simulink model "RoboticArm"  (R2023b)
settings: Solver=ode23t  StartTime=0.0  StopTime=100  RelTol=1e-3
model workspace: external: MATLAB File D:\Projects\RoboticArm\RoboticArm_DataFile1.m (data not in the file)
undefined symbols (not defined in the file or in its folder): dfdbk, dFilt, nfdbk, nFilt, smiData, ST, X, Y, Z
libraries: sm_lib x180, fl_lib x129, nesl_utility x69, ee_lib x39, slpidlib x25, simulink x18, SignalEditorBlockLib x1
(part 3 of 7)

== system RoboticArm/Control System3/Subsystem3 ==
  signal : Inport
  Abs : Abs  SaturateOnIntegerOverflow=off
  Fcn : Fcn  Expr=u(1)<0
  Gain : Gain  Gain=5
  "[0...5]" : Saturate  UpperLimit=5  LowerLimit=0
  duty : Outport
  rev : Outport  Port=2
  wires:
  signal/1 -> Fcn/1, Abs/1
  Abs/1 -> "[0...5]"/1
  Fcn/1 -> Gain/1
  Gain/1 -> rev/1
  "[0...5]"/1 -> duty/1

== system RoboticArm/Control System3/Subsystem4 ==
  signal : Inport
  Abs : Abs  SaturateOnIntegerOverflow=off
  Fcn : Fcn  Expr=u(1)<0
  Gain : Gain  Gain=5
  "[0...5]" : Saturate  UpperLimit=5  LowerLimit=0
  duty : Outport
  rev : Outport  Port=2
  wires:
  "[0...5]"/1 -> duty/1
  Gain/1 -> rev/1
  Fcn/1 -> Gain/1
  Abs/1 -> "[0...5]"/1
  signal/1 -> Abs/1, Fcn/1

== system RoboticArm/Control System3/Subsystem5 ==
  signal : Inport
  Abs : Abs  SaturateOnIntegerOverflow=off
  Fcn : Fcn  Expr=u(1)<0
  Gain : Gain  Gain=5
  "[0...5]" : Saturate  UpperLimit=5  LowerLimit=0
  duty : Outport
  rev : Outport  Port=2
  wires:
  signal/1 -> Fcn/1, Abs/1
  Abs/1 -> "[0...5]"/1
  Fcn/1 -> Gain/1
  Gain/1 -> rev/1
  "[0...5]"/1 -> duty/1

== system RoboticArm/Control System3/Subsystem6 ==
  signal : Inport
  Abs : Abs  SaturateOnIntegerOverflow=off
  Fcn : Fcn  Expr=u(1)<0
  Gain : Gain  Gain=5
  "[0...5]" : Saturate  UpperLimit=5  LowerLimit=0
  duty : Outport
  rev : Outport  Port=2
  wires:
  "[0...5]"/1 -> duty/1
  Gain/1 -> rev/1
  Fcn/1 -> Gain/1
  Abs/1 -> "[0...5]"/1
  signal/1 -> Abs/1, Fcn/1

== system RoboticArm/Control System3/Transfer Function ==
  Fdbk : Inport
  Bus Creator6 : BusCreator  Inputs=6
  Bus Selector2 : BusSelector  OutputSignals=tAngle,bAngle,fAngle,wAngle,hAngle,gAngle
  Constant1 : Constant  Value=pi/2
  Discrete Transfer Fcn{,1..5} (6 alike) : DiscreteTransferFcn  Numerator=nFilt  Denominator=dFilt  SampleTime=ST
  Sum1 : Sum  Inputs=|+-
  Angles : Outport
  wires:
  Sum1/1 -> Discrete Transfer Fcn1/1
  Discrete Transfer Fcn2/1 -> Bus Creator6/3  "fAngle"
  Discrete Transfer Fcn/1 -> Bus Creator6/1  "tAngle"
  Discrete Transfer Fcn3/1 -> Bus Creator6/4  "wAngle"
  Discrete Transfer Fcn4/1 -> Bus Creator6/5  "hAngle"
  Fdbk/1 -> Bus Selector2/1
  Discrete Transfer Fcn5/1 -> Bus Creator6/6  "gAngle"
  Discrete Transfer Fcn1/1 -> Bus Creator6/2  "bAngle"
  Constant1/1 -> Sum1/2
  Bus Selector2/2 -> Sum1/1  "<bAngle>"
  Bus Selector2/4 -> Discrete Transfer Fcn3/1  "<wAngle>"
  Bus Selector2/1 -> Discrete Transfer Fcn/1  "<tAngle>"
  Bus Creator6/1 -> Angles/1
  Bus Selector2/3 -> Discrete Transfer Fcn2/1  "<fAngle>"
  Bus Selector2/6 -> Discrete Transfer Fcn5/1  "<gAngle>"
  Bus Selector2/5 -> Discrete Transfer Fcn4/1  "<hAngle>"

== system RoboticArm/Controller1/Signal Conditioning ==
  note: Anti-aliasing filters
  fddk : Inport
  Bus Creator3 : BusCreator  Inputs=6
  Bus Selector : BusSelector  OutputSignals=tAngle,bAngle,fAngle,wAngle,hAngle,gAngle
  Discrete Transfer Fcn{,1..5} (6 alike) : DiscreteTransferFcn  Numerator=nFilt  Denominator=dFilt  SampleTime=ST
  IC : Constant  Value=pi
  Sum : Sum  Inputs=|+-
  angles (rad) : Outport  VectorParamsAs1DForOutWhenUnconnected=off
  wires:
  IC/1 -> Sum/2
  Sum/1 -> Discrete Transfer Fcn1/1
  Bus Selector/2 -> Sum/1  "<bAngle>"
  Bus Selector/6 -> Discrete Transfer Fcn5/1  "<gAngle>"
  Bus Selector/5 -> Discrete Transfer Fcn4/1  "<hAngle>"
  Discrete Transfer Fcn5/1 -> Bus Creator3/6  "gAngle"
  Discrete Transfer Fcn4/1 -> Bus Creator3/5  "hAngle"
  Bus Creator3/1 -> angles (rad)/1
  Discrete Transfer Fcn3/1 -> Bus Creator3/4  "wAngle"
  Discrete Transfer Fcn2/1 -> Bus Creator3/3  "fAngle"
  Bus Selector/3 -> Discrete Transfer Fcn2/1  "<fAngle>"
  Bus Selector/4 -> Discrete Transfer Fcn3/1  "<wAngle>"
  Bus Selector/1 -> Discrete Transfer Fcn/1  "<tAngle>"
  fddk/1 -> Bus Selector/1
  Discrete Transfer Fcn/1 -> Bus Creator3/1  "tAngle"
  Discrete Transfer Fcn1/1 -> Bus Creator3/2  "bAngle"

== system RoboticArm/Controller1/bicepCMD ==
  Vcmd : Inport
  Vbrk : Inport  Port=2
  Abs : Abs  SaturateOnIntegerOverflow=off
  Fcn : Fcn  Expr=u(1)<0
  Gain : Gain  Gain=5
  "[0...5]" : Saturate  UpperLimit=100  LowerLimit=0
  "[0...5] " : Saturate  UpperLimit=5  LowerLimit=0
  Duty : Outport  VectorParamsAs1DForOutWhenUnconnected=off
  REV : Outport  Port=2  VectorParamsAs1DForOutWhenUnconnected=off
  BRK : Outport  Port=3  VectorParamsAs1DForOutWhenUnconnected=off
  wires:
  "[0...5] "/1 -> BRK/1
  Vbrk/1 -> "[0...5] "/1
  Vcmd/1 -> Fcn/1, Abs/1
  Abs/1 -> "[0...5]"/1
  Fcn/1 -> Gain/1
  "[0...5]"/1 -> Duty/1
  Gain/1 -> REV/1

== system RoboticArm/Controller1/forearmCMD ==
  Vcmd : Inport
  Vbrk : Inport  Port=2
  Abs : Abs  SaturateOnIntegerOverflow=off
  Fcn : Fcn  Expr=u(1)<0
  Gain : Gain  Gain=5
  "[0...5]" : Saturate  UpperLimit=5  LowerLimit=0
  "[0...5] " : Saturate  UpperLimit=5  LowerLimit=0
  Duty : Outport  VectorParamsAs1DForOutWhenUnconnected=off
  REV : Outport  Port=2  VectorParamsAs1DForOutWhenUnconnected=off
  BRK : Outport  Port=3  VectorParamsAs1DForOutWhenUnconnected=off
  wires:
  Gain/1 -> REV/1
  "[0...5]"/1 -> Duty/1
  Fcn/1 -> Gain/1
  Abs/1 -> "[0...5]"/1
  Vcmd/1 -> Abs/1, Fcn/1
  Vbrk/1 -> "[0...5] "/1
  "[0...5] "/1 -> BRK/1

== system RoboticArm/Controller1/gripperCMD ==
  Vcmd : Inport
  Vbrk : Inport  Port=2
  Abs : Abs  SaturateOnIntegerOverflow=off
  Fcn : Fcn  Expr=u(1)<0
  Gain : Gain  Gain=5
  "[0...5]" : Saturate  UpperLimit=5  LowerLimit=0
  "[0...5] " : Saturate  UpperLimit=5  LowerLimit=0
  Duty : Outport  VectorParamsAs1DForOutWhenUnconnected=off
  REV : Outport  Port=2  VectorParamsAs1DForOutWhenUnconnected=off
  BRK : Outport  Port=3  VectorParamsAs1DForOutWhenUnconnected=off
  wires:
  Gain/1 -> REV/1
  "[0...5]"/1 -> Duty/1
  Fcn/1 -> Gain/1
  Abs/1 -> "[0...5]"/1
  Vcmd/1 -> Abs/1, Fcn/1
  Vbrk/1 -> "[0...5] "/1
  "[0...5] "/1 -> BRK/1

== system RoboticArm/Controller1/handCMD ==
  Vcmd : Inport
  Vbrk : Inport  Port=2
  Abs : Abs  SaturateOnIntegerOverflow=off
  Fcn : Fcn  Expr=u(1)<0
  Gain : Gain  Gain=5
  "[0...5]" : Saturate  UpperLimit=5  LowerLimit=0
  "[0...5] " : Saturate  UpperLimit=5  LowerLimit=0
  Duty : Outport  VectorParamsAs1DForOutWhenUnconnected=off
  REV : Outport  Port=2  VectorParamsAs1DForOutWhenUnconnected=off
  BRK : Outport  Port=3  VectorParamsAs1DForOutWhenUnconnected=off
  wires:
  "[0...5] "/1 -> BRK/1
  Vbrk/1 -> "[0...5] "/1
  Vcmd/1 -> Fcn/1, Abs/1
  Abs/1 -> "[0...5]"/1
  Fcn/1 -> Gain/1
  "[0...5]"/1 -> Duty/1
  Gain/1 -> REV/1

== system RoboticArm/Controller1/turntableCMD ==
  Vcmd : Inport
  Vbrk : Inport  Port=2
  Abs : Abs  SaturateOnIntegerOverflow=off
  Fcn : Fcn  Expr=u(1)<0
  Gain : Gain  Gain=5
  "[0...5]" : Saturate  UpperLimit=5  LowerLimit=0
  "[0...5] " : Saturate  UpperLimit=5  LowerLimit=0
  Duty : Outport  VectorParamsAs1DForOutWhenUnconnected=off
  REV : Outport  Port=2  VectorParamsAs1DForOutWhenUnconnected=off
  BRK : Outport  Port=3  VectorParamsAs1DForOutWhenUnconnected=off
  wires:
  Gain/1 -> REV/1
  "[0...5]"/1 -> Duty/1
  Fcn/1 -> Gain/1
  Abs/1 -> "[0...5]"/1
  Vcmd/1 -> Abs/1, Fcn/1
  Vbrk/1 -> "[0...5] "/1
  "[0...5] "/1 -> BRK/1

== system RoboticArm/Controller1/wristCMD ==
  Vcmd : Inport
  Vbrk : Inport  Port=2
  Abs : Abs  SaturateOnIntegerOverflow=off
  Fcn : Fcn  Expr=u(1)<0
  Gain : Gain  Gain=5
  "[0...5]" : Saturate  UpperLimit=5  LowerLimit=0
  "[0...5] " : Saturate  UpperLimit=5  LowerLimit=0
  Duty : Outport  VectorParamsAs1DForOutWhenUnconnected=off
  REV : Outport  Port=2  VectorParamsAs1DForOutWhenUnconnected=off
  BRK : Outport  Port=3  VectorParamsAs1DForOutWhenUnconnected=off
  wires:
  Gain/1 -> REV/1
  "[0...5]"/1 -> Duty/1
  Fcn/1 -> Gain/1
  Abs/1 -> "[0...5]"/1
  Vcmd/1 -> Abs/1, Fcn/1
  Vbrk/1 -> "[0...5] "/1
  "[0...5] "/1 -> BRK/1

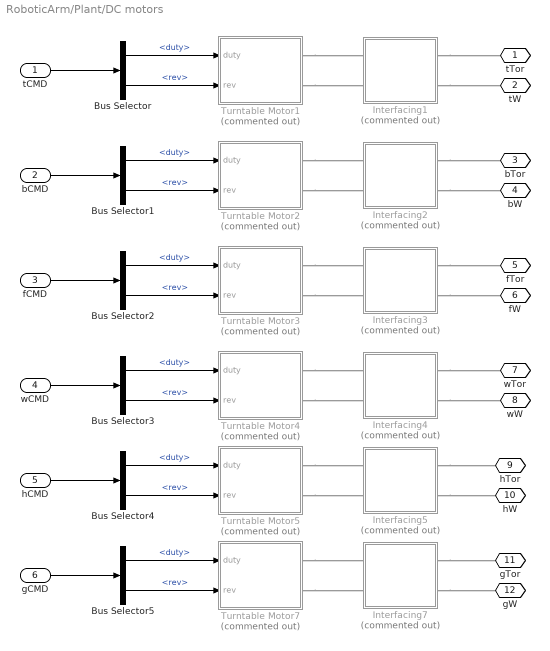
== system RoboticArm/Plant/DC motors ==
  tCMD : Inport
  bCMD : Inport  Port=2
  fCMD : Inport  Port=3
  wCMD : Inport  Port=4
  hCMD : Inport  Port=5
  gCMD : Inport  Port=6
  Bus Selector{,1..5} (6 alike) : BusSelector  OutputSignals=duty,rev
  Interfacing1 : Subsystem  Commented=on
      mask Display: image('interface-4.png');
  Interfacing2 : Subsystem  Commented=on
      mask Display: image('interface-4.png');
  Interfacing3 : Subsystem  Commented=on
      mask Display: image('interface-4.png');
  Interfacing4 : Subsystem  Commented=on
      mask Display: image('interface-4.png');
  Interfacing5 : Subsystem  Commented=on
      mask Display: image('interface-4.png');
  Interfacing7 : Subsystem  Commented=on
      mask Display: image('interface-4.png');
  Turntable Motor1 : Subsystem  Commented=on
      mask Display: image('servo1.jpg');
  Turntable Motor2 : Subsystem  Commented=on
      mask Display: image('servo1.jpg');
  Turntable Motor3 : Subsystem  Commented=on
      mask Display: image('servo1.jpg');
  Turntable Motor4 : Subsystem  Commented=on
      mask Display: image('servo1.jpg');
  Turntable Motor5 : Subsystem  Commented=on
      mask Display: image('servo1.jpg');
  Turntable Motor7 : Subsystem  Commented=on
      mask Display: image('servo1.jpg');
  tTor : PMIOPort  Side=Right
  tW : PMIOPort  Port=2  Side=Right
  bTor : PMIOPort  Port=3  Side=Right
  bW : PMIOPort  Port=4  Side=Right
  fTor : PMIOPort  Port=5  Side=Right
  fW : PMIOPort  Port=6  Side=Right
  wTor : PMIOPort  Port=7  Side=Right
  wW : PMIOPort  Port=8  Side=Right
  hTor : PMIOPort  Port=9  Side=Right
  hW : PMIOPort  Port=10  Side=Right
  gTor : PMIOPort  Port=11  Side=Right
  gW : PMIOPort  Port=12  Side=Right
  wires:
  wCMD/1 -> Bus Selector3/1
  bCMD/1 -> Bus Selector1/1
  gCMD/1 -> Bus Selector5/1
  fCMD/1 -> Bus Selector2/1
  tCMD/1 -> Bus Selector/1
  hCMD/1 -> Bus Selector4/1
  Bus Selector/1 -> Turntable Motor1/1(duty)  "<duty>"
  Bus Selector/2 -> Turntable Motor1/2(rev)  "<rev>"
  Bus Selector1/1 -> Turntable Motor2/1(duty)  "<duty>"
  Bus Selector1/2 -> Turntable Motor2/2(rev)  "<rev>"
  Bus Selector2/2 -> Turntable Motor3/2(rev)  "<rev>"
  Bus Selector2/1 -> Turntable Motor3/1(duty)  "<duty>"
  Bus Selector3/1 -> Turntable Motor4/1(duty)  "<duty>"
  Bus Selector3/2 -> Turntable Motor4/2(rev)  "<rev>"
  Bus Selector4/1 -> Turntable Motor5/1(duty)  "<duty>"
  Bus Selector4/2 -> Turntable Motor5/2(rev)  "<rev>"
  Bus Selector5/1 -> Turntable Motor7/1(duty)  "<duty>"
  Bus Selector5/2 -> Turntable Motor7/2(rev)  "<rev>"
  connections:
  Interfacing1/RConn2 -- tW/RConn1
  Interfacing1/RConn1 -- tTor/RConn1
  Interfacing2/RConn1 -- bTor/RConn1
  Interfacing2/RConn2 -- bW/RConn1
  Interfacing3/RConn2 -- fW/RConn1
  Interfacing3/RConn1 -- fTor/RConn1
  Interfacing4/RConn1 -- wTor/RConn1
  Interfacing4/RConn2 -- wW/RConn1
  Interfacing5/RConn2 -- hW/RConn1
  Interfacing5/RConn1 -- hTor/RConn1
  Interfacing7/RConn1 -- gTor/RConn1
  Interfacing7/RConn2 -- gW/RConn1
  Turntable Motor1/RConn2 -- Interfacing1/LConn2
  Turntable Motor1/RConn1 -- Interfacing1/LConn1
  Turntable Motor2/RConn1 -- Interfacing2/LConn1
  Turntable Motor2/RConn2 -- Interfacing2/LConn2
  Turntable Motor3/RConn2 -- Interfacing3/LConn2
  Turntable Motor3/RConn1 -- Interfacing3/LConn1
  Turntable Motor4/RConn1 -- Interfacing4/LConn1
  Turntable Motor4/RConn2 -- Interfacing4/LConn2
  Turntable Motor5/RConn2 -- Interfacing5/LConn2
  Turntable Motor5/RConn1 -- Interfacing5/LConn1
  Turntable Motor7/RConn1 -- Interfacing7/LConn1
  Turntable Motor7/RConn2 -- Interfacing7/LConn2

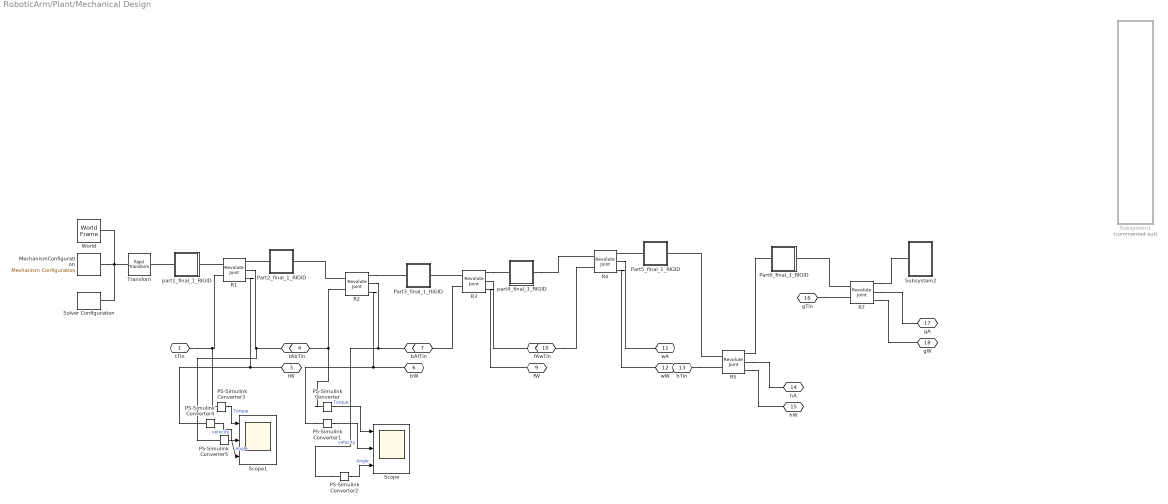
== system RoboticArm/Plant/Mechanical Design ==
  MechanismConfiguration : sm_lib/Utilities/Mechanism Configuration  UniformGravity=Constant  GravityVector=[0 -9.81 0]  GravityVectorUnits=m/s^2  LinearizationDelta=0.001  JointModeTransitionNonlinearIterations=2
  PS-Simulink Converter{,1..5} (6 alike) : nesl_utility/PS-Simulink Converter  PhysicalDomain=network_engine_domain  SubClassName=ps_output  LeftPortType=input  RightPortType=output  PseudoPeriodic=off  Frequencies=[]  VectorFormat=inherit  Unit=inherit  AffineConversion=off
  Part2_final_1_RIGID : Subsystem
  Part3_final_1_RIGID : Subsystem
  Part5_final_1_RIGID : Subsystem
  Part6_final_1_RIGID : Subsystem
  R{1..5,7} (6 alike) : sm_lib/Joints/Revolute Joint  JointMode=Normal  SenseConstraintForce=off  SenseConstraintForceX=off  SenseConstraintForceY=off  SenseConstraintForceZ=off  SenseConstraintTorque=off  SenseConstraintTorqueX=off  SenseConstraintTorqueY=off  SenseConstraintTorqueZ=off  SenseTotalForce=off  SenseTotalForceX=off  SenseTotalForceY=off  SenseTotalForceZ=off  SenseTotalTorque=off  SenseTotalTorqueX=off  SenseTotalTorqueY=off  SenseTotalTorqueZ=off  CompositeWrenchDir=FollowerOnBase  CompositeWrenchFrame=BaseFrame  EquilibriumPosition=0  EquilibriumPositionUnits=rad  SpringStiffness=0  SpringStiffnessUnits=m*N/rad  DampingCoefficient=0  DampingCoefficientUnits=m*s*N/rad  TorqueActuationMode=InputTorque  MotionActuationMode=ComputedMotion  SensePosition=on  SenseVelocity=on  SenseAcceleration=off  SenseTorqueForce=off  SenseLowerLimitTorqueForce=off  SenseUpperLimitTorqueForce=off  LowerLimitSpecify=off  LowerLimitBound=-90  LowerLimitBoundUnits=deg  LowerLimitStiffness=1e4  LowerLimitStiffnessUnits=N*m/deg  LowerLimitDamping=10  LowerLimitDampingUnits=N*m/(deg/s)  LowerLimitTransitionRegionWidth=0.1  LowerLimitTransitionRegionWidthUnits=deg  UpperLimitSpecify=off  UpperLimitBound=90  UpperLimitBoundUnits=deg  UpperLimitStiffness=1e4  UpperLimitStiffnessUnits=N*m/deg  UpperLimitDamping=10  UpperLimitDampingUnits=N*m/(deg/s)  UpperLimitTransitionRegionWidth=0.1  UpperLimitTransitionRegionWidthUnits=deg  PositionTargetSpecify=on  PositionTargetPriority=High  PositionTargetValue=0  PositionTargetValueUnits=deg  VelocityTargetSpecify=on  VelocityTargetPriority=High  VelocityTargetValue=0  VelocityTargetValueUnits=deg/s
  Scope : Scope  NumInputPorts=3
  Scope1 : Scope  NumInputPorts=3
  Solver Configuration : nesl_utility/Solver Configuration  PhysicalDomain=network_engine_domain  SubClassName=solver  LeftPortType=input  RightPortType=generic  Tones=[]  Harmonics=[]  SimulateNoise=off  Profile=off  UseLocalSampling=off  EnableSwitchedLinearOptims=on  FrequencyDomain=off  UseCCode=off  RelTol=0.001  AbsTol=1e-06  MinStep=1e-09  ToWorkspace=off  RevertToSquareIcSolve=off  NumHomotopyIterations=100  PhasorMode=off  PhasorModeNumHarmonics=1  ConsistencySolver=NEWTON_FTOL  IndexReductionMethod=DerivativeReplacement  DoDC=off  ResidualTolerance=1e-09  ConsistencyTolSource=GLOBAL  ConsistencyAbsTol=0.001  ConsistencyRelTol=0.001  ConsistencyTolFactor=0.001  UseLocalSolver=off  LocalSolverChoice=NE_BACKWARD_EULER_ADVANCER  ResolveIndetEquations=on  FunctionEvalNumThread=1  LocalSolverSampleTime=0.001  DoFixedCost=off  MaxNonlinIter=3  MaxModeIter=2  ComputeImpulses=off  ImpulseIterations=2  LinearAlgebra=Sparse  LinearAlgebraNumThread=0  EquationFormulation=NE_TIME_EF  DelaysMemoryBudget=1024  AutomaticFiltering=on  FilteringTimeConstant=0.001  PartitionStorageMethod=AS_NEEDED  PartitionMemoryBudget=1024  PartitionMethod=FAST  MultibodyUseLocalSolver=off  MultibodyLocalSolverChoice=ODE1  MultibodyLocalSolverSampleTime=0.001
  Subsystem1 : Subsystem  Commented=on
  Subsystem2 : Subsystem
  Transforn : sm_lib/Frames and Transforms/Rigid Transform  TranslationMethod=None  TranslationStandardOffset=0  TranslationStandardOffsetUnits=m  TranslationStandardAxis=+Z  TranslationCartesianOffset=[0 0 0]  TranslationCartesianOffsetUnits=m  TranslationROffset=0  TranslationROffsetUnits=m  TranslationZOffset=0  TranslationZOffsetUnits=m  TranslationThetaOffset=0  TranslationThetaOffsetUnits=deg  RotationMethod=None  RotationAngleUnits=deg  RotationStandardAxis=+Z  RotationAngle=0.0  RotationArbitraryAxis=[0 0 1]  FollAlignAxisA=+X  BaseAlignAxisA=+Y  FollAlignAxisB=+Y  BaseAlignAxisB=+Z  RotationSequenceAxes=FollowerAxes  RotationSequence=XYX  RotationSequenceAngles=[0 0 0]  RotationSequenceAnglesUnits=deg  RotationMatrix=[1 0 0; 0 1 0; 0 0 1]  Quaternion=[1 0 0 0]
  World : sm_lib/Frames and Transforms/World Frame
  part1_final_1_RIGID : Subsystem
  part4_final_1_RIGID : Subsystem
  tTin : PMIOPort  Side=Left
  tA : PMIOPort  Port=2  Side=Right
  tW : PMIOPort  Port=3  Side=Left
  bTin : PMIOPort  Port=4  Side=Left
  bA : PMIOPort  Port=5  Side=Right
  bW : PMIOPort  Port=6  Side=Left
  fTin : PMIOPort  Port=7  Side=Left
  fA : PMIOPort  Port=8  Side=Right
  fW : PMIOPort  Port=9  Side=Left
  wTin : PMIOPort  Port=10  Side=Left
  wA : PMIOPort  Port=11  Side=Right
  wW : PMIOPort  Port=12  Side=Left
  hTin : PMIOPort  Port=13  Side=Left
  hA : PMIOPort  Port=14  Side=Right
  hW : PMIOPort  Port=15  Side=Left
  gTin : PMIOPort  Port=16  Side=Left
  gA : PMIOPort  Port=17  Side=Right
  gW : PMIOPort  Port=18  Side=Left
  wires:
  PS-Simulink Converter2/1 -> Scope/3  "Angle"
  PS-Simulink Converter5/1 -> Scope1/3  "Angle"
  PS-Simulink Converter/1 -> Scope/1  "Torque"
  PS-Simulink Converter4/1 -> Scope1/2  "velocity"
  PS-Simulink Converter1/1 -> Scope/2  "velocity"
  PS-Simulink Converter3/1 -> Scope1/1  "Torque"
  connections:
  R1/RConn2 -- tA/RConn1 -- PS-Simulink Converter5/LConn1
  PS-Simulink Converter1/LConn1 -- bW/RConn1 -- R2/RConn3
  PS-Simulink Converter/LConn1 -- bTin/RConn1 -- R2/LConn2
  R1/LConn2 -- tTin/RConn1 -- PS-Simulink Converter3/LConn1
  PS-Simulink Converter2/LConn1 -- bA/RConn1 -- R2/RConn2
  Solver Configuration/RConn1 -- World/RConn1 -- Transforn/LConn1 -- MechanismConfiguration/RConn1
  PS-Simulink Converter4/LConn1 -- tW/RConn1 -- R1/RConn3
  R7/RConn3 -- gW/RConn1
  R2/LConn1 -- Part2_final_1_RIGID/RConn1
  R5/RConn3 -- hW/RConn1
  R7/LConn1 -- Part6_final_1_RIGID/RConn1
  R5/RConn2 -- hA/RConn1
  wTin/RConn1 -- R4/LConn2
  R5/LConn1 -- Part5_final_1_RIGID/RConn1
  R3/RConn3 -- fW/RConn1
  R4/RConn3 -- wW/RConn1
  hTin/RConn1 -- R5/LConn2
  R3/LConn2 -- fTin/RConn1
  R7/RConn2 -- gA/RConn1
  R4/RConn2 -- wA/RConn1
  R3/RConn2 -- fA/RConn1
  gTin/RConn1 -- R7/LConn2
  Part2_final_1_RIGID/LConn1 -- R1/RConn1
  R7/RConn1 -- Subsystem2/LConn1
  R3/LConn1 -- Part3_final_1_RIGID/RConn1
  Part5_final_1_RIGID/LConn1 -- R4/RConn1
  part1_final_1_RIGID/LConn1 -- Transforn/RConn1
  R3/RConn1 -- part4_final_1_RIGID/LConn1
  part4_final_1_RIGID/RConn1 -- R4/LConn1
  R2/RConn1 -- Part3_final_1_RIGID/LConn1
  R1/LConn1 -- part1_final_1_RIGID/RConn1
  Part6_final_1_RIGID/LConn1 -- R5/RConn1

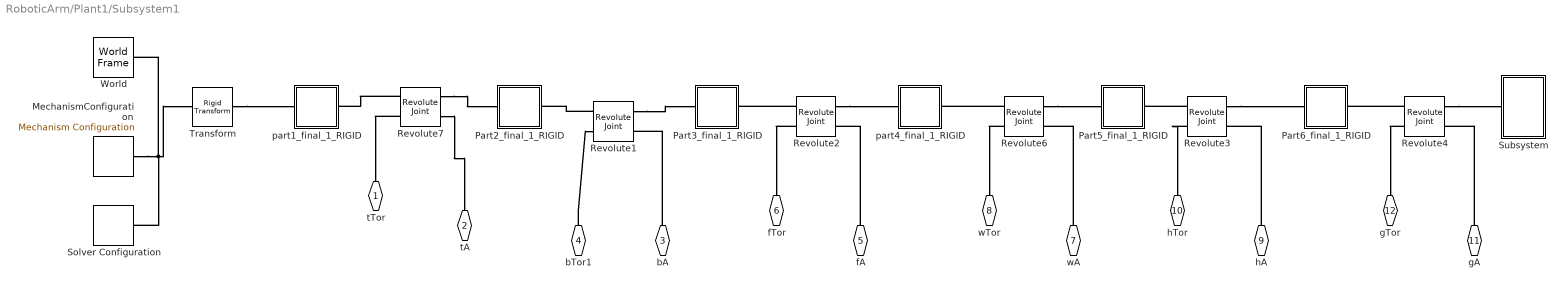
== system RoboticArm/Plant1/Subsystem1 ==
  MechanismConfiguration : sm_lib/Utilities/Mechanism Configuration  UniformGravity=Constant  GravityVector=[0 -9.80665 0]  GravityVectorUnits=m/s^2  LinearizationDelta=0.001  JointModeTransitionNonlinearIterations=2
  Part2_final_1_RIGID : Subsystem
  Part3_final_1_RIGID : Subsystem
  Part5_final_1_RIGID : Subsystem
  Part6_final_1_RIGID : Subsystem
  Revolute{1..4,6..7} (6 alike) : sm_lib/Joints/Revolute Joint  JointMode=Normal  SenseConstraintForce=off  SenseConstraintForceX=off  SenseConstraintForceY=off  SenseConstraintForceZ=off  SenseConstraintTorque=off  SenseConstraintTorqueX=off  SenseConstraintTorqueY=off  SenseConstraintTorqueZ=off  SenseTotalForce=off  SenseTotalForceX=off  SenseTotalForceY=off  SenseTotalForceZ=off  SenseTotalTorque=off  SenseTotalTorqueX=off  SenseTotalTorqueY=off  SenseTotalTorqueZ=off  CompositeWrenchDir=FollowerOnBase  CompositeWrenchFrame=BaseFrame  EquilibriumPosition=0  EquilibriumPositionUnits=deg  SpringStiffness=0  SpringStiffnessUnits=N*m/deg  DampingCoefficient=0  DampingCoefficientUnits=N*m/(deg/s)  TorqueActuationMode=ComputedTorque  MotionActuationMode=InputMotion  SensePosition=on  SenseVelocity=off  SenseAcceleration=off  SenseTorqueForce=off  SenseLowerLimitTorqueForce=off  SenseUpperLimitTorqueForce=off  LowerLimitSpecify=off  LowerLimitBound=-90  LowerLimitBoundUnits=deg  LowerLimitStiffness=1e4  LowerLimitStiffnessUnits=N*m/deg  LowerLimitDamping=10  LowerLimitDampingUnits=N*m/(deg/s)  LowerLimitTransitionRegionWidth=0.1  LowerLimitTransitionRegionWidthUnits=deg  UpperLimitSpecify=off  UpperLimitBound=90  UpperLimitBoundUnits=deg  UpperLimitStiffness=1e4  UpperLimitStiffnessUnits=N*m/deg  UpperLimitDamping=10  UpperLimitDampingUnits=N*m/(deg/s)  UpperLimitTransitionRegionWidth=0.1  UpperLimitTransitionRegionWidthUnits=deg  PositionTargetSpecify=on  PositionTargetPriority=Low  PositionTargetValue=smiData.RevoluteJoint(7).Rz.Pos  PositionTargetValueUnits=deg  VelocityTargetSpecify=off  VelocityTargetPriority=High  VelocityTargetValue=0  VelocityTargetValueUnits=deg/s
  Solver Configuration : nesl_utility/Solver Configuration  PhysicalDomain=network_engine_domain  SubClassName=solver  LeftPortType=input  RightPortType=generic  Tones=[]  Harmonics=[]  SimulateNoise=off  Profile=off  UseLocalSampling=off  EnableSwitchedLinearOptims=on  FrequencyDomain=off  UseCCode=off  RelTol=0.001  AbsTol=0.001  MinStep=1e-09  ToWorkspace=off  RevertToSquareIcSolve=off  NumHomotopyIterations=100  PhasorMode=off  PhasorModeNumHarmonics=1  ConsistencySolver=NEWTON_XTOL_AFTER_FTOL  IndexReductionMethod=DerivativeReplacement  DoDC=off  ResidualTolerance=1e-09  ConsistencyTolSource=GLOBAL  ConsistencyAbsTol=0.001  ConsistencyRelTol=0.001  ConsistencyTolFactor=0.001  UseLocalSolver=off  LocalSolverChoice=NE_BACKWARD_EULER_ADVANCER  ResolveIndetEquations=on  FunctionEvalNumThread=1  LocalSolverSampleTime=0.001  DoFixedCost=off  MaxNonlinIter=3  MaxModeIter=2  ComputeImpulses=off  ImpulseIterations=2  LinearAlgebra=auto  LinearAlgebraNumThread=0  EquationFormulation=NE_TIME_EF  DelaysMemoryBudget=1024  AutomaticFiltering=on  FilteringTimeConstant=0.001  PartitionStorageMethod=AS_NEEDED  PartitionMemoryBudget=1024  PartitionMethod=ROBUST  MultibodyUseLocalSolver=off  MultibodyLocalSolverChoice=ODE1  MultibodyLocalSolverSampleTime=0.001
  Subsystem : Subsystem
  Transform : sm_lib/Frames and Transforms/Rigid Transform  TranslationMethod=Cartesian  TranslationStandardOffset=0  TranslationStandardOffsetUnits=m  TranslationStandardAxis=+Z  TranslationCartesianOffset=smiData.RigidTransform(17).translation  TranslationCartesianOffsetUnits=mm  TranslationROffset=0  TranslationROffsetUnits=m  TranslationZOffset=0  TranslationZOffsetUnits=m  TranslationThetaOffset=0  TranslationThetaOffsetUnits=deg  RotationMethod=ArbitraryAxis  RotationAngleUnits=rad  RotationStandardAxis=+Z  RotationAngle=smiData.RigidTransform(17).angle  RotationArbitraryAxis=smiData.RigidTransform(17).axis  FollAlignAxisA=+X  BaseAlignAxisA=+Y  FollAlignAxisB=+Y  BaseAlignAxisB=+Z  RotationSequenceAxes=FollowerAxes  RotationSequence=XYX  RotationSequenceAngles=[0 0 0]  RotationSequenceAnglesUnits=deg  RotationMatrix=[1 0 0; 0 1 0; 0 0 1]  Quaternion=[1 0 0 0]
  World : sm_lib/Frames and Transforms/World Frame
  part1_final_1_RIGID : Subsystem
  part4_final_1_RIGID : Subsystem
  tTor : PMIOPort  Side=Left
  tA : PMIOPort  Port=2  Side=Right
  bA : PMIOPort  Port=3  Side=Right
  bTor1 : PMIOPort  Port=4  Side=Left
  fA : PMIOPort  Port=5  Side=Right
  fTor : PMIOPort  Port=6  Side=Left
  wA : PMIOPort  Port=7  Side=Right
  wTor : PMIOPort  Port=8  Side=Left
  hA : PMIOPort  Port=9  Side=Right
  hTor : PMIOPort  Port=10  Side=Left
  gA : PMIOPort  Port=11  Side=Right
  gTor : PMIOPort  Port=12  Side=Left
  connections:
  Revolute4/LConn1 -- Part6_final_1_RIGID/RConn1
  gA/RConn1 -- Revolute4/RConn2
  bTor1/RConn1 -- Revolute1/LConn2
  Revolute6/RConn1 -- Part5_final_1_RIGID/LConn1
  bA/RConn1 -- Revolute1/RConn2
  Revolute2/LConn2 -- fTor/RConn1
  hA/RConn1 -- Revolute3/RConn2
  Revolute4/LConn2 -- gTor/RConn1
  Revolute1/LConn1 -- Part2_final_1_RIGID/RConn1
  Revolute6/LConn2 -- wTor/RConn1
  Revolute4/RConn1 -- Subsystem/LConn1
  Revolute1/RConn1 -- Part3_final_1_RIGID/LConn1
  Transform/RConn1 -- part1_final_1_RIGID/LConn1
  Revolute7/LConn1 -- part1_final_1_RIGID/RConn1
  Revolute3/LConn1 -- Part5_final_1_RIGID/RConn1
  Revolute3/RConn1 -- Part6_final_1_RIGID/LConn1
  Revolute3/LConn2 -- hTor/RConn1
  World/RConn1 -- Solver Configuration/RConn1 -- MechanismConfiguration/RConn1 -- Transform/LConn1
  Revolute2/RConn1 -- part4_final_1_RIGID/LConn1
  Revolute7/LConn2 -- tTor/RConn1
  fA/RConn1 -- Revolute2/RConn2
  Revolute7/RConn1 -- Part2_final_1_RIGID/LConn1
  Revolute7/RConn2 -- tA/RConn1
  wA/RConn1 -- Revolute6/RConn2
  Revolute6/LConn1 -- part4_final_1_RIGID/RConn1
  Revolute2/LConn1 -- Part3_final_1_RIGID/RConn1

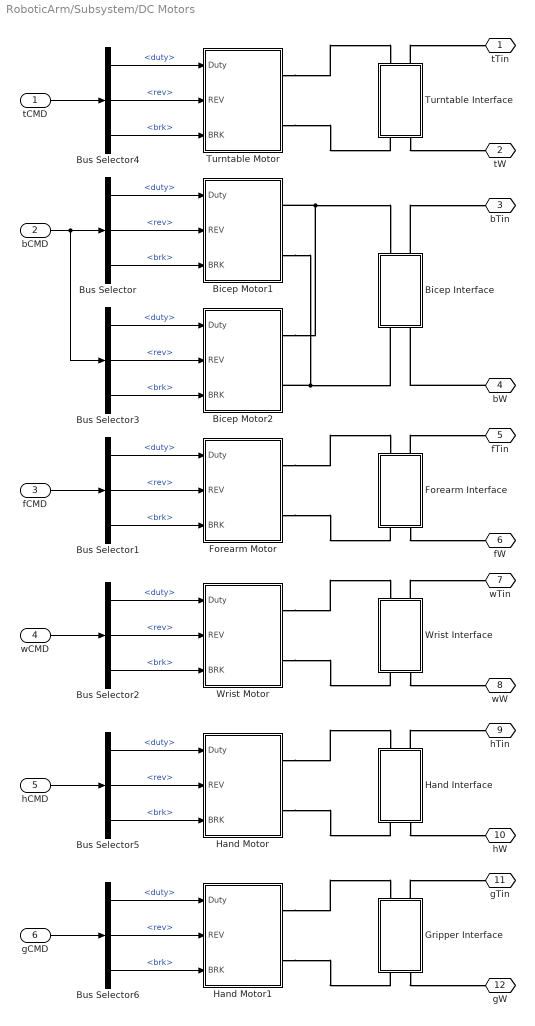
== system RoboticArm/Subsystem/DC Motors ==
  tCMD : Inport
  bCMD : Inport  Port=2
  fCMD : Inport  Port=3
  wCMD : Inport  Port=4
  hCMD : Inport  Port=5
  gCMD : Inport  Port=6
  Bicep Interface : Subsystem
  Bicep Motor1 : Subsystem
      mask Display: image('Servo.jpg')
  Bicep Motor2 : Subsystem
      mask Display: image('Servo.jpg')
  Bus Selector{,1..6} (7 alike) : BusSelector  OutputSignals=duty,rev,brk
  Forearm Interface : Subsystem
  Forearm Motor : Subsystem
      mask Display: image('Servo.jpg')
  Gripper Interface : Subsystem
  Hand Interface : Subsystem
  Hand Motor : Subsystem
      mask Display: image('Servo.jpg')
  Hand Motor1 : Subsystem
      mask Display: image('Servo.jpg')
  Turntable Interface : Subsystem
  Turntable Motor : Subsystem
      mask Display: image('Servo.jpg')
  Wrist Interface : Subsystem
  Wrist Motor : Subsystem
      mask Display: image('Servo.jpg')
  tTin : PMIOPort  Side=Right
  tW : PMIOPort  Port=2  Side=Right
  bTin : PMIOPort  Port=3  Side=Right
  bW : PMIOPort  Port=4  Side=Right
  fTin : PMIOPort  Port=5  Side=Right
  fW : PMIOPort  Port=6  Side=Right
  wTin : PMIOPort  Port=7  Side=Right
  wW : PMIOPort  Port=8  Side=Right
  hTin : PMIOPort  Port=9  Side=Right
  hW : PMIOPort  Port=10  Side=Right
  gTin : PMIOPort  Port=11  Side=Right
  gW : PMIOPort  Port=12  Side=Right
  wires:
  bCMD/1 -> Bus Selector/1, Bus Selector3/1
  Bus Selector/1 -> Bicep Motor1/1(Duty)  "<duty>"
  Bus Selector/2 -> Bicep Motor1/2(REV)  "<rev>"
  Bus Selector/3 -> Bicep Motor1/3(BRK)  "<brk>"
  fCMD/1 -> Bus Selector1/1
  Bus Selector1/1 -> Forearm Motor/1(Duty)  "<duty>"
  Bus Selector1/2 -> Forearm Motor/2(REV)  "<rev>"
  Bus Selector1/3 -> Forearm Motor/3(BRK)  "<brk>"
  Bus Selector3/1 -> Bicep Motor2/1(Duty)  "<duty>"
  Bus Selector3/2 -> Bicep Motor2/2(REV)  "<rev>"
  Bus Selector3/3 -> Bicep Motor2/3(BRK)  "<brk>"
  wCMD/1 -> Bus Selector2/1
  Bus Selector2/1 -> Wrist Motor/1(Duty)  "<duty>"
  Bus Selector2/2 -> Wrist Motor/2(REV)  "<rev>"
  Bus Selector2/3 -> Wrist Motor/3(BRK)  "<brk>"
  tCMD/1 -> Bus Selector4/1
  Bus Selector4/1 -> Turntable Motor/1(Duty)  "<duty>"
  Bus Selector4/2 -> Turntable Motor/2(REV)  "<rev>"
  Bus Selector4/3 -> Turntable Motor/3(BRK)  "<brk>"
  hCMD/1 -> Bus Selector5/1
  Bus Selector5/1 -> Hand Motor/1(Duty)  "<duty>"
  Bus Selector5/2 -> Hand Motor/2(REV)  "<rev>"
  Bus Selector5/3 -> Hand Motor/3(BRK)  "<brk>"
  gCMD/1 -> Bus Selector6/1
  Bus Selector6/1 -> Hand Motor1/1(Duty)  "<duty>"
  Bus Selector6/2 -> Hand Motor1/2(REV)  "<rev>"
  Bus Selector6/3 -> Hand Motor1/3(BRK)  "<brk>"
  connections:
  Bicep Motor2/RConn1 -- Bicep Motor1/RConn1 -- Bicep Interface/LConn1
  Bicep Motor1/RConn2 -- Bicep Motor2/RConn2 -- Bicep Interface/RConn1
  Forearm Motor/RConn2 -- Forearm Interface/RConn1
  Forearm Motor/RConn1 -- Forearm Interface/LConn1
  Forearm Interface/RConn2 -- fW/RConn1
  Bicep Interface/LConn2 -- bTin/RConn1
  Forearm Interface/LConn2 -- fTin/RConn1
  bW/RConn1 -- Bicep Interface/RConn2
  Wrist Motor/RConn2 -- Wrist Interface/RConn1
  Wrist Interface/LConn2 -- wTin/RConn1
  Wrist Motor/RConn1 -- Wrist Interface/LConn1
  Wrist Interface/RConn2 -- wW/RConn1
  Turntable Interface/LConn2 -- tTin/RConn1
  Turntable Motor/RConn1 -- Turntable Interface/LConn1
  Turntable Motor/RConn2 -- Turntable Interface/RConn1
  Turntable Interface/RConn2 -- tW/RConn1
  Hand Interface/RConn2 -- hW/RConn1
  Hand Motor/RConn1 -- Hand Interface/LConn1
  Hand Interface/LConn2 -- hTin/RConn1
  Hand Motor/RConn2 -- Hand Interface/RConn1
  Hand Motor1/RConn2 -- Gripper Interface/RConn1
  Gripper Interface/RConn2 -- gW/RConn1
  Hand Motor1/RConn1 -- Gripper Interface/LConn1
  Gripper Interface/LConn2 -- gTin/RConn1

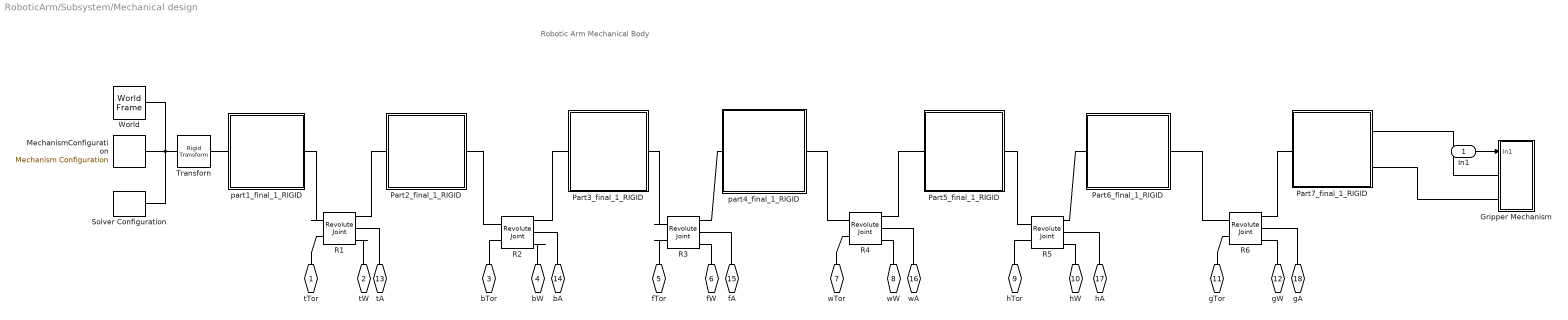
== system RoboticArm/Subsystem/Mechanical design ==
  note: Robotic Arm Mechanical Body
  In1 : Inport
  Gripper Mechanism : Subsystem
  MechanismConfiguration : sm_lib/Utilities/Mechanism Configuration  UniformGravity=Constant  GravityVector=[0 -9.81 0]  GravityVectorUnits=m/s^2  LinearizationDelta=0.001  JointModeTransitionNonlinearIterations=2
  Part2_final_1_RIGID : Subsystem
      mask Display: image('Screenshot 2024-04-15 210704.png');
  Part3_final_1_RIGID : Subsystem
      mask Display: image('Screenshot 2024-04-15 210823.png');
  Part5_final_1_RIGID : Subsystem
      mask Display: image('Screenshot 2024-04-15 210946.png');
  Part6_final_1_RIGID : Subsystem
      mask Display: image('Screenshot 2024-04-15 211030.png');
  Part7_final_1_RIGID : Subsystem
      mask Display: image('Screenshot 2024-04-15 211044.png');
  R{1..6} (6 alike) : sm_lib/Joints/Revolute Joint  JointMode=Normal  SenseConstraintForce=off  SenseConstraintForceX=off  SenseConstraintForceY=off  SenseConstraintForceZ=off  SenseConstraintTorque=off  SenseConstraintTorqueX=off  SenseConstraintTorqueY=off  SenseConstraintTorqueZ=off  SenseTotalForce=off  SenseTotalForceX=off  SenseTotalForceY=off  SenseTotalForceZ=off  SenseTotalTorque=off  SenseTotalTorqueX=off  SenseTotalTorqueY=off  SenseTotalTorqueZ=off  CompositeWrenchDir=FollowerOnBase  CompositeWrenchFrame=BaseFrame  EquilibriumPosition=0  EquilibriumPositionUnits=rad  SpringStiffness=0  SpringStiffnessUnits=m*N/rad  DampingCoefficient=0  DampingCoefficientUnits=m*s*N/rad  TorqueActuationMode=InputTorque  MotionActuationMode=ComputedMotion  SensePosition=on  SenseVelocity=on  SenseAcceleration=off  SenseTorqueForce=off  SenseLowerLimitTorqueForce=off  SenseUpperLimitTorqueForce=off  LowerLimitSpecify=off  LowerLimitBound=-90  LowerLimitBoundUnits=deg  LowerLimitStiffness=1e4  LowerLimitStiffnessUnits=N*m/deg  LowerLimitDamping=10  LowerLimitDampingUnits=N*m/(deg/s)  LowerLimitTransitionRegionWidth=0.1  LowerLimitTransitionRegionWidthUnits=deg  UpperLimitSpecify=off  UpperLimitBound=90  UpperLimitBoundUnits=deg  UpperLimitStiffness=1e4  UpperLimitStiffnessUnits=N*m/deg  UpperLimitDamping=10  UpperLimitDampingUnits=N*m/(deg/s)  UpperLimitTransitionRegionWidth=0.1  UpperLimitTransitionRegionWidthUnits=deg  PositionTargetSpecify=on  PositionTargetPriority=High  PositionTargetValue=0  PositionTargetValueUnits=deg  VelocityTargetSpecify=on  VelocityTargetPriority=High  VelocityTargetValue=0  VelocityTargetValueUnits=deg/s
  Solver Configuration : nesl_utility/Solver Configuration  PhysicalDomain=network_engine_domain  SubClassName=solver  LeftPortType=input  RightPortType=generic  Tones=[]  Harmonics=[]  SimulateNoise=off  Profile=off  UseLocalSampling=off  EnableSwitchedLinearOptims=on  FrequencyDomain=off  UseCCode=off  RelTol=0.001  AbsTol=1e-06  MinStep=1e-09  ToWorkspace=off  RevertToSquareIcSolve=off  NumHomotopyIterations=100  PhasorMode=off  PhasorModeNumHarmonics=1  ConsistencySolver=NEWTON_FTOL  IndexReductionMethod=DerivativeReplacement  DoDC=off  ResidualTolerance=1e-09  ConsistencyTolSource=GLOBAL  ConsistencyAbsTol=0.001  ConsistencyRelTol=0.001  ConsistencyTolFactor=0.001  UseLocalSolver=off  LocalSolverChoice=NE_BACKWARD_EULER_ADVANCER  ResolveIndetEquations=on  FunctionEvalNumThread=1  LocalSolverSampleTime=0.001  DoFixedCost=off  MaxNonlinIter=3  MaxModeIter=2  ComputeImpulses=off  ImpulseIterations=2  LinearAlgebra=Sparse  LinearAlgebraNumThread=0  EquationFormulation=NE_TIME_EF  DelaysMemoryBudget=1024  AutomaticFiltering=on  FilteringTimeConstant=0.001  PartitionStorageMethod=AS_NEEDED  PartitionMemoryBudget=1024  PartitionMethod=FAST  MultibodyUseLocalSolver=off  MultibodyLocalSolverChoice=ODE1  MultibodyLocalSolverSampleTime=0.001
  Transforn : sm_lib/Frames and Transforms/Rigid Transform  TranslationMethod=None  TranslationStandardOffset=0  TranslationStandardOffsetUnits=m  TranslationStandardAxis=+Z  TranslationCartesianOffset=[0 0 0]  TranslationCartesianOffsetUnits=m  TranslationROffset=0  TranslationROffsetUnits=m  TranslationZOffset=0  TranslationZOffsetUnits=m  TranslationThetaOffset=0  TranslationThetaOffsetUnits=deg  RotationMethod=None  RotationAngleUnits=deg  RotationStandardAxis=+Z  RotationAngle=0.0  RotationArbitraryAxis=[0 0 1]  FollAlignAxisA=+X  BaseAlignAxisA=+Y  FollAlignAxisB=+Y  BaseAlignAxisB=+Z  RotationSequenceAxes=FollowerAxes  RotationSequence=XYX  RotationSequenceAngles=[0 0 0]  RotationSequenceAnglesUnits=deg  RotationMatrix=[1 0 0; 0 1 0; 0 0 1]  Quaternion=[1 0 0 0]
  World : sm_lib/Frames and Transforms/World Frame
  part1_final_1_RIGID : Subsystem
      mask Display: image('Screenshot 2024-04-15 210633.png');
  part4_final_1_RIGID : Subsystem
      mask Display: image('Screenshot 2024-04-15 210901.png');
  tTor : PMIOPort  Side=Left
  tW : PMIOPort  Port=2  Side=Left
  bTor : PMIOPort  Port=3  Side=Left
  bW : PMIOPort  Port=4  Side=Left
  fTor : PMIOPort  Port=5  Side=Left
  fW : PMIOPort  Port=6  Side=Left
  wTor : PMIOPort  Port=7  Side=Left
  wW : PMIOPort  Port=8  Side=Left
  hTor : PMIOPort  Port=9  Side=Left
  hW : PMIOPort  Port=10  Side=Left
  gTor : PMIOPort  Port=11  Side=Left
  gW : PMIOPort  Port=12  Side=Left
  tA : PMIOPort  Port=13  Side=Right
  bA : PMIOPort  Port=14  Side=Right
  fA : PMIOPort  Port=15  Side=Right
  wA : PMIOPort  Port=16  Side=Right
  hA : PMIOPort  Port=17  Side=Right
  gA : PMIOPort  Port=18  Side=Right
  wires:
  In1/1 -> Gripper Mechanism/1(In1)
  connections:
  R3/RConn2 -- fA/RConn1
  R3/LConn1 -- Part3_final_1_RIGID/RConn1
  Transforn/LConn1 -- Solver Configuration/RConn1 -- MechanismConfiguration/RConn1 -- World/RConn1
  R1/RConn3 -- tW/RConn1
  R2/RConn3 -- bW/RConn1
  wTor/RConn1 -- R4/LConn2
  R2/RConn2 -- bA/RConn1
  R6/RConn3 -- gW/RConn1
  tTor/RConn1 -- R1/LConn2
  Part5_final_1_RIGID/LConn1 -- R4/RConn1
  R4/RConn3 -- wW/RConn1
  hTor/RConn1 -- R5/LConn2
  R5/LConn1 -- Part5_final_1_RIGID/RConn1
  R1/LConn1 -- part1_final_1_RIGID/RConn1
  part1_final_1_RIGID/LConn1 -- Transforn/RConn1
  R5/RConn3 -- hW/RConn1
  R2/LConn1 -- Part2_final_1_RIGID/RConn1
  Part7_final_1_RIGID/LConn1 -- R6/RConn1
  part4_final_1_RIGID/RConn1 -- R4/LConn1
  gTor/RConn1 -- R6/LConn2
  R2/LConn2 -- bTor/RConn1
  Part6_final_1_RIGID/LConn1 -- R5/RConn1
  R5/RConn2 -- hA/RConn1
  R6/RConn2 -- gA/RConn1
  R3/LConn2 -- fTor/RConn1
  R3/RConn1 -- part4_final_1_RIGID/LConn1
  R6/LConn1 -- Part6_final_1_RIGID/RConn1
  R4/RConn2 -- wA/RConn1
  Part7_final_1_RIGID/RConn1 -- Gripper Mechanism/LConn1
  R2/RConn1 -- Part3_final_1_RIGID/LConn1
  Part2_final_1_RIGID/LConn1 -- R1/RConn1
  R3/RConn3 -- fW/RConn1
  Part7_final_1_RIGID/RConn2 -- Gripper Mechanism/LConn2
  R1/RConn2 -- tA/RConn1

== system RoboticArm/Subsystem1/Transfer Function ==
  Fdbk : Inport
  Bus Creator6 : BusCreator  Inputs=6
  Bus Selector2 : BusSelector  OutputSignals=tAngle,bAngle,fAngle,wAngle,hAngle,gAngle
  Constant1 : Constant  Value=pi/2
  Discrete Transfer Fcn{,1..5} (6 alike) : DiscreteTransferFcn  Numerator=nfdbk  Denominator=dfdbk  SampleTime=ST
  Sum1 : Sum  Inputs=|+-
  Angles : Outport
  wires:
  Bus Selector2/5 -> Discrete Transfer Fcn4/1  "<hAngle>"
  Bus Selector2/6 -> Discrete Transfer Fcn5/1  "<gAngle>"
  Bus Selector2/3 -> Discrete Transfer Fcn2/1  "<fAngle>"
  Bus Creator6/1 -> Angles/1
  Bus Selector2/1 -> Discrete Transfer Fcn/1  "<tAngle>"
  Bus Selector2/4 -> Discrete Transfer Fcn3/1  "<wAngle>"
  Bus Selector2/2 -> Sum1/1  "<bAngle>"
  Constant1/1 -> Sum1/2
  Discrete Transfer Fcn1/1 -> Bus Creator6/2  "bAngle"
  Discrete Transfer Fcn5/1 -> Bus Creator6/6  "gAngle"
  Fdbk/1 -> Bus Selector2/1
  Discrete Transfer Fcn4/1 -> Bus Creator6/5  "hAngle"
  Discrete Transfer Fcn3/1 -> Bus Creator6/4  "wAngle"
  Discrete Transfer Fcn/1 -> Bus Creator6/1  "tAngle"
  Discrete Transfer Fcn2/1 -> Bus Creator6/3  "fAngle"
  Sum1/1 -> Discrete Transfer Fcn1/1

== system RoboticArm/Plant/DC motors/Interfacing1 ==
  Ideal Angular Velocity Source : fl_lib/Mechanical/Mechanical Sources/Ideal Angular Velocity Source
  Ideal Torque Sensor : fl_lib/Mechanical/Mechanical Sensors/Ideal Torque Sensor
  R : PMIOPort  Side=Left
  C : PMIOPort  Port=2  Side=Left
  T : PMIOPort  Port=3  Side=Right
  W : PMIOPort  Port=4  Side=Right
  connections:
  W/RConn1 -- Ideal Angular Velocity Source/RConn1
  Ideal Torque Sensor/RConn1 -- Ideal Angular Velocity Source/LConn1
  Ideal Torque Sensor/RConn2 -- T/RConn1
  Ideal Angular Velocity Source/RConn2 -- C/RConn1
  R/RConn1 -- Ideal Torque Sensor/LConn1

== system RoboticArm/Plant/DC motors/Interfacing2 ==
  Ideal Angular Velocity Source : fl_lib/Mechanical/Mechanical Sources/Ideal Angular Velocity Source
  Ideal Torque Sensor : fl_lib/Mechanical/Mechanical Sensors/Ideal Torque Sensor
  R : PMIOPort  Side=Left
  C : PMIOPort  Port=2  Side=Left
  T : PMIOPort  Port=3  Side=Right
  W : PMIOPort  Port=4  Side=Right
  connections:
  R/RConn1 -- Ideal Torque Sensor/LConn1
  Ideal Angular Velocity Source/RConn2 -- C/RConn1
  Ideal Torque Sensor/RConn2 -- T/RConn1
  Ideal Torque Sensor/RConn1 -- Ideal Angular Velocity Source/LConn1
  W/RConn1 -- Ideal Angular Velocity Source/RConn1

== system RoboticArm/Plant/DC motors/Interfacing3 ==
  Ideal Angular Velocity Source : fl_lib/Mechanical/Mechanical Sources/Ideal Angular Velocity Source
  Ideal Torque Sensor : fl_lib/Mechanical/Mechanical Sensors/Ideal Torque Sensor
  R : PMIOPort  Side=Left
  C : PMIOPort  Port=2  Side=Left
  T : PMIOPort  Port=3  Side=Right
  W : PMIOPort  Port=4  Side=Right
  connections:
  W/RConn1 -- Ideal Angular Velocity Source/RConn1
  Ideal Torque Sensor/RConn1 -- Ideal Angular Velocity Source/LConn1
  Ideal Torque Sensor/RConn2 -- T/RConn1
  Ideal Angular Velocity Source/RConn2 -- C/RConn1
  R/RConn1 -- Ideal Torque Sensor/LConn1

== system RoboticArm/Plant/DC motors/Interfacing4 ==
  Ideal Angular Velocity Source : fl_lib/Mechanical/Mechanical Sources/Ideal Angular Velocity Source
  Ideal Torque Sensor : fl_lib/Mechanical/Mechanical Sensors/Ideal Torque Sensor
  R : PMIOPort  Side=Left
  C : PMIOPort  Port=2  Side=Left
  T : PMIOPort  Port=3  Side=Right
  W : PMIOPort  Port=4  Side=Right
  connections:
  R/RConn1 -- Ideal Torque Sensor/LConn1
  Ideal Angular Velocity Source/RConn2 -- C/RConn1
  Ideal Torque Sensor/RConn2 -- T/RConn1
  Ideal Torque Sensor/RConn1 -- Ideal Angular Velocity Source/LConn1
  W/RConn1 -- Ideal Angular Velocity Source/RConn1

== system RoboticArm/Plant/DC motors/Interfacing5 ==
  Ideal Angular Velocity Source : fl_lib/Mechanical/Mechanical Sources/Ideal Angular Velocity Source
  Ideal Torque Sensor : fl_lib/Mechanical/Mechanical Sensors/Ideal Torque Sensor
  R : PMIOPort  Side=Left
  C : PMIOPort  Port=2  Side=Left
  T : PMIOPort  Port=3  Side=Right
  W : PMIOPort  Port=4  Side=Right
  connections:
  W/RConn1 -- Ideal Angular Velocity Source/RConn1
  Ideal Torque Sensor/RConn1 -- Ideal Angular Velocity Source/LConn1
  Ideal Torque Sensor/RConn2 -- T/RConn1
  Ideal Angular Velocity Source/RConn2 -- C/RConn1
  R/RConn1 -- Ideal Torque Sensor/LConn1

== system RoboticArm/Plant/DC motors/Interfacing7 ==
  Ideal Angular Velocity Source : fl_lib/Mechanical/Mechanical Sources/Ideal Angular Velocity Source
  Ideal Torque Sensor : fl_lib/Mechanical/Mechanical Sensors/Ideal Torque Sensor
  R : PMIOPort  Side=Left
  C : PMIOPort  Port=2  Side=Left
  T : PMIOPort  Port=3  Side=Right
  W : PMIOPort  Port=4  Side=Right
  connections:
  R/RConn1 -- Ideal Torque Sensor/LConn1
  Ideal Angular Velocity Source/RConn2 -- C/RConn1
  Ideal Torque Sensor/RConn2 -- T/RConn1
  Ideal Torque Sensor/RConn1 -- Ideal Angular Velocity Source/LConn1
  W/RConn1 -- Ideal Angular Velocity Source/RConn1

== system RoboticArm/Plant/DC motors/Turntable Motor1 ==
  duty : Inport
  rev : Inport  Port=2
  DC Motor : ee_lib/Electromechanical/Brushed Motors/DC Motor  field_option=ee.enum.field_option.pm  Rf=100 Ohm  Lf=1 H  Laf=0.15 H  If0=0 A  parameterization=ee.enum.dcparam_option.circuit_param  Ra=4.9994 Ohm  La=0.00031645 H  emf_or_torque=ee.enum.emf_or_torque.ki  Kv=0.072e-3 V/rpm  Ki=0.47777 N*m/A  T_stall=0.24e-3 N*m  w_max=19100 rpm  w_rated=15000 rpm  P_rated=0.08 W  V_rated=1.5 V  lam_param=ee.enum.lam_param.damping  i_noload=0 A  V_i_noload=1.5 V  J=0 cm^2*g  lam=0.92143 N*m*s/rad  speed0=0 rpm  enable_fault_armature=simscape.enum.onoff.off  rev_faulted=1 / 3  G_faulted_armature=1e-5 S  fault_trigger_armature=ee.enum.faults.faultTrigger.temporal  t_fault_armature=1 s  max_permissible_current_armature=inf A  t_fail_on_current_armature=1 s  enable_fault_field=simscape.enum.onoff.off  G_faulted_field=1e-5 S  fault_trigger_field=ee.enum.faults.faultTrigger.temporal  t_fault_field=1 s  max_permissible_current_field=inf A  t_fail_on_current_field=1 s  fault_action=simscape.enum.assert.action.none  alpha=3.93e-3 1/K  Tmeas=25 degC  thermal_mass=100 J/K  initial_temperature=25 degC
  Electrical Reference : fl_lib/Electrical/Electrical Elements/Electrical Reference
  Mechanical Rotational Reference : fl_lib/Mechanical/Rotational Elements/Mechanical Rotational Reference
  Power Amplifier : Subsystem
      mask Display: image('H bridge.jpg');
  R : PMIOPort  Side=Right
  C : PMIOPort  Port=2  Side=Right
  wires:
  rev/1 -> Power Amplifier/2(rev)
  duty/1 -> Power Amplifier/1(duty)
  connections:
  DC Motor/RConn1 -- Power Amplifier/RConn2 -- Electrical Reference/LConn1
  DC Motor/RConn2 -- Mechanical Rotational Reference/LConn1 -- C/RConn1
  DC Motor/LConn2 -- R/RConn1
  DC Motor/LConn1 -- Power Amplifier/RConn1

== system RoboticArm/Plant/DC motors/Turntable Motor2 ==
  duty : Inport
  rev : Inport  Port=2
  DC Motor : ee_lib/Electromechanical/Brushed Motors/DC Motor  field_option=ee.enum.field_option.pm  Rf=100 Ohm  Lf=1 H  Laf=0.15 H  If0=0 A  parameterization=ee.enum.dcparam_option.circuit_param  Ra=4.9994 Ohm  La=0.00031645 H  emf_or_torque=ee.enum.emf_or_torque.ki  Kv=0.072e-3 V/rpm  Ki=0.47777 N*m/A  T_stall=0.24e-3 N*m  w_max=19100 rpm  w_rated=15000 rpm  P_rated=0.08 W  V_rated=1.5 V  lam_param=ee.enum.lam_param.damping  i_noload=0 A  V_i_noload=1.5 V  J=0 cm^2*g  lam=0.92143 N*m*s/rad  speed0=0 rpm  enable_fault_armature=simscape.enum.onoff.off  rev_faulted=1 / 3  G_faulted_armature=1e-5 S  fault_trigger_armature=ee.enum.faults.faultTrigger.temporal  t_fault_armature=1 s  max_permissible_current_armature=inf A  t_fail_on_current_armature=1 s  enable_fault_field=simscape.enum.onoff.off  G_faulted_field=1e-5 S  fault_trigger_field=ee.enum.faults.faultTrigger.temporal  t_fault_field=1 s  max_permissible_current_field=inf A  t_fail_on_current_field=1 s  fault_action=simscape.enum.assert.action.none  alpha=3.93e-3 1/K  Tmeas=25 degC  thermal_mass=100 J/K  initial_temperature=25 degC
  Electrical Reference : fl_lib/Electrical/Electrical Elements/Electrical Reference
  Mechanical Rotational Reference : fl_lib/Mechanical/Rotational Elements/Mechanical Rotational Reference
  Power Amplifier : Subsystem
      mask Display: image('H bridge.jpg');
  R : PMIOPort  Side=Right
  C : PMIOPort  Port=2  Side=Right
  wires:
  duty/1 -> Power Amplifier/1(duty)
  rev/1 -> Power Amplifier/2(rev)
  connections:
  DC Motor/LConn1 -- Power Amplifier/RConn1
  DC Motor/LConn2 -- R/RConn1
  C/RConn1 -- Mechanical Rotational Reference/LConn1 -- DC Motor/RConn2
  Electrical Reference/LConn1 -- Power Amplifier/RConn2 -- DC Motor/RConn1

== system RoboticArm/Plant/DC motors/Turntable Motor3 ==
  duty : Inport
  rev : Inport  Port=2
  DC Motor : ee_lib/Electromechanical/Brushed Motors/DC Motor  field_option=ee.enum.field_option.pm  Rf=100 Ohm  Lf=1 H  Laf=0.15 H  If0=0 A  parameterization=ee.enum.dcparam_option.circuit_param  Ra=4.9994 Ohm  La=0.00031645 H  emf_or_torque=ee.enum.emf_or_torque.ki  Kv=0.072e-3 V/rpm  Ki=0.47777 N*m/A  T_stall=0.24e-3 N*m  w_max=19100 rpm  w_rated=15000 rpm  P_rated=0.08 W  V_rated=1.5 V  lam_param=ee.enum.lam_param.damping  i_noload=0 A  V_i_noload=1.5 V  J=0 cm^2*g  lam=0.92143 N*m*s/rad  speed0=0 rpm  enable_fault_armature=simscape.enum.onoff.off  rev_faulted=1 / 3  G_faulted_armature=1e-5 S  fault_trigger_armature=ee.enum.faults.faultTrigger.temporal  t_fault_armature=1 s  max_permissible_current_armature=inf A  t_fail_on_current_armature=1 s  enable_fault_field=simscape.enum.onoff.off  G_faulted_field=1e-5 S  fault_trigger_field=ee.enum.faults.faultTrigger.temporal  t_fault_field=1 s  max_permissible_current_field=inf A  t_fail_on_current_field=1 s  fault_action=simscape.enum.assert.action.none  alpha=3.93e-3 1/K  Tmeas=25 degC  thermal_mass=100 J/K  initial_temperature=25 degC
  Electrical Reference : fl_lib/Electrical/Electrical Elements/Electrical Reference
  Mechanical Rotational Reference : fl_lib/Mechanical/Rotational Elements/Mechanical Rotational Reference
  Power Amplifier : Subsystem
      mask Display: image('H bridge.jpg');
  R : PMIOPort  Side=Right
  C : PMIOPort  Port=2  Side=Right
  wires:
  rev/1 -> Power Amplifier/2(rev)
  duty/1 -> Power Amplifier/1(duty)
  connections:
  DC Motor/RConn1 -- Power Amplifier/RConn2 -- Electrical Reference/LConn1
  DC Motor/RConn2 -- Mechanical Rotational Reference/LConn1 -- C/RConn1
  DC Motor/LConn2 -- R/RConn1
  DC Motor/LConn1 -- Power Amplifier/RConn1

== system RoboticArm/Plant/DC motors/Turntable Motor4 ==
  duty : Inport
  rev : Inport  Port=2
  DC Motor : ee_lib/Electromechanical/Brushed Motors/DC Motor  field_option=ee.enum.field_option.pm  Rf=100 Ohm  Lf=1 H  Laf=0.15 H  If0=0 A  parameterization=ee.enum.dcparam_option.circuit_param  Ra=4.9994 Ohm  La=0.00031645 H  emf_or_torque=ee.enum.emf_or_torque.ki  Kv=0.072e-3 V/rpm  Ki=0.47777 N*m/A  T_stall=0.24e-3 N*m  w_max=19100 rpm  w_rated=15000 rpm  P_rated=0.08 W  V_rated=1.5 V  lam_param=ee.enum.lam_param.damping  i_noload=0 A  V_i_noload=1.5 V  J=0 cm^2*g  lam=0.92143 N*m*s/rad  speed0=0 rpm  enable_fault_armature=simscape.enum.onoff.off  rev_faulted=1 / 3  G_faulted_armature=1e-5 S  fault_trigger_armature=ee.enum.faults.faultTrigger.temporal  t_fault_armature=1 s  max_permissible_current_armature=inf A  t_fail_on_current_armature=1 s  enable_fault_field=simscape.enum.onoff.off  G_faulted_field=1e-5 S  fault_trigger_field=ee.enum.faults.faultTrigger.temporal  t_fault_field=1 s  max_permissible_current_field=inf A  t_fail_on_current_field=1 s  fault_action=simscape.enum.assert.action.none  alpha=3.93e-3 1/K  Tmeas=25 degC  thermal_mass=100 J/K  initial_temperature=25 degC
  Electrical Reference : fl_lib/Electrical/Electrical Elements/Electrical Reference
  Mechanical Rotational Reference : fl_lib/Mechanical/Rotational Elements/Mechanical Rotational Reference
  Power Amplifier : Subsystem
      mask Display: image('H bridge.jpg');
  R : PMIOPort  Side=Right
  C : PMIOPort  Port=2  Side=Right
  wires:
  duty/1 -> Power Amplifier/1(duty)
  rev/1 -> Power Amplifier/2(rev)
  connections:
  DC Motor/LConn1 -- Power Amplifier/RConn1
  DC Motor/LConn2 -- R/RConn1
  C/RConn1 -- Mechanical Rotational Reference/LConn1 -- DC Motor/RConn2
  Electrical Reference/LConn1 -- Power Amplifier/RConn2 -- DC Motor/RConn1

== system RoboticArm/Plant/DC motors/Turntable Motor5 ==
  duty : Inport
  rev : Inport  Port=2
  DC Motor : ee_lib/Electromechanical/Brushed Motors/DC Motor  field_option=ee.enum.field_option.pm  Rf=100 Ohm  Lf=1 H  Laf=0.15 H  If0=0 A  parameterization=ee.enum.dcparam_option.circuit_param  Ra=4.9994 Ohm  La=0.00031645 H  emf_or_torque=ee.enum.emf_or_torque.ki  Kv=0.072e-3 V/rpm  Ki=0.47777 N*m/A  T_stall=0.24e-3 N*m  w_max=19100 rpm  w_rated=15000 rpm  P_rated=0.08 W  V_rated=1.5 V  lam_param=ee.enum.lam_param.damping  i_noload=0 A  V_i_noload=1.5 V  J=0 cm^2*g  lam=0.92143 N*m*s/rad  speed0=0 rpm  enable_fault_armature=simscape.enum.onoff.off  rev_faulted=1 / 3  G_faulted_armature=1e-5 S  fault_trigger_armature=ee.enum.faults.faultTrigger.temporal  t_fault_armature=1 s  max_permissible_current_armature=inf A  t_fail_on_current_armature=1 s  enable_fault_field=simscape.enum.onoff.off  G_faulted_field=1e-5 S  fault_trigger_field=ee.enum.faults.faultTrigger.temporal  t_fault_field=1 s  max_permissible_current_field=inf A  t_fail_on_current_field=1 s  fault_action=simscape.enum.assert.action.none  alpha=3.93e-3 1/K  Tmeas=25 degC  thermal_mass=100 J/K  initial_temperature=25 degC
  Electrical Reference : fl_lib/Electrical/Electrical Elements/Electrical Reference
  Mechanical Rotational Reference : fl_lib/Mechanical/Rotational Elements/Mechanical Rotational Reference
  Power Amplifier : Subsystem
      mask Display: image('H bridge.jpg');
  R : PMIOPort  Side=Right
  C : PMIOPort  Port=2  Side=Right
  wires:
  rev/1 -> Power Amplifier/2(rev)
  duty/1 -> Power Amplifier/1(duty)
  connections:
  DC Motor/RConn1 -- Power Amplifier/RConn2 -- Electrical Reference/LConn1
  DC Motor/RConn2 -- Mechanical Rotational Reference/LConn1 -- C/RConn1
  DC Motor/LConn2 -- R/RConn1
  DC Motor/LConn1 -- Power Amplifier/RConn1
